simulink model "rlocus_tf"  (R2025b)
settings: Solver=VariableStepAuto  StartTime=0.0  StopTime=10.0  RelTol=1e-3
values from neighbouring files (symbols this model uses):
  den = [tau   1]    [Copy_of_LQR_ctrl.m]    (also in LQR_ctrl.m)
  num = [1]    [Copy_of_LQR_ctrl.m]    (also in LQR_ctrl.m)
  poles = [p_c; -0.01; -0.02]    [Rlocus_ctrl.m]    (also in pole_placement_ctrl.m = [ -500 ; -62 ; -2+2.7j ; -2-2.7j ])
settings Model: Creator=Abhi  LastModifiedBy=Abhi

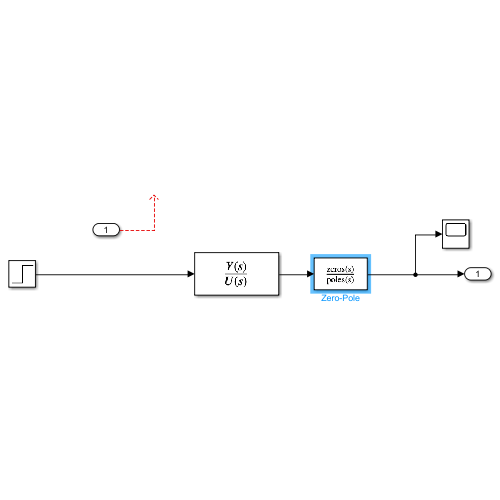
[thumbnail: Simulink's stored preview of the top-level diagram]
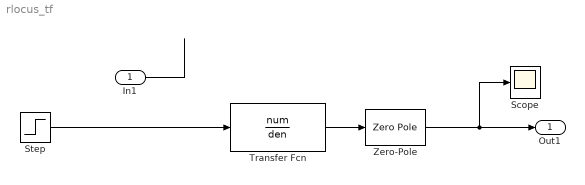
== system rlocus_tf ==
  In1 : Inport
  Scope : Scope
      settings: ActiveDisplayYMinimum=-3.7036527384776512E+78  ActiveDisplayYMaximum=4.1151697094196117E+77
  Step : Step  SampleTime=0
  Transfer Fcn : TransferFcn  Numerator=num  Denominator=den  ContinuousStateAttributes='x_b'
  Zero-Pole : ZeroPole  Zeros=[]  Poles=poles  ContinuousStateAttributes='x_b'
  Out1 : Outport
  wires:
  Transfer Fcn/1 -> Zero-Pole/1
  Zero-Pole/1 -> Scope/1, Out1/1
  Step/1 -> Transfer Fcn/1
  In1/1 -> ?
